simulink subsystem "model_inductance_L2"  (R2024a)
settings: Solver=VariableStepAuto  StartTime=0.0  StopTime=10.0  RelTol=1e-3
undefined symbols (not defined in the file): d, r
settings Model: Creator=Bocchio  LastModifiedBy=Bocchio

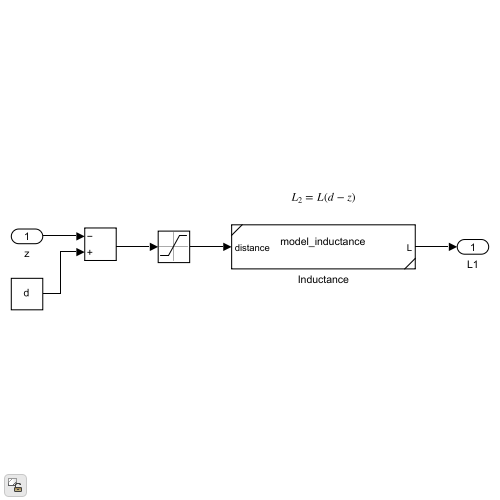
[thumbnail: Simulink's stored preview of the top-level diagram]
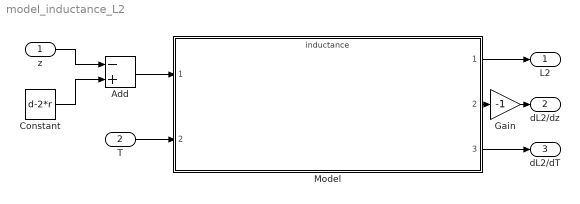
== system model_inductance_L2 ==
  z : Inport
  T : Inport  Port=2
  Add : Sum  Inputs=-+
  Constant : Constant  Value=d-2*r
  Gain : Gain  Gain=-1
  Model : ModelReference  ModelNameDialog=inductance.slx  SimulationMode=Normal  ModelReferenceVersion=1.2
  L2 : Outport
  dL2/dz : Outport  Port=2
  dL2/dT : Outport  Port=3
  wires:
  z/1 -> Add/1
  Constant/1 -> Add/2
  Model/3 -> dL2/dT/1
  Add/1 -> Model/1
  T/1 -> Model/2
  Model/1 -> L2/1
  Model/2 -> Gain/1
  Gain/1 -> dL2/dz/1
